simulink library "tbdc"  (Simulink 8.1)
settings: Solver=ode1  StartTime=0.0  StopTime=Inf  FixedStep=0.001  RelTol=1e-3
PostLoadFcn:
  | , if any(exist('dsrtsu_mdlpostloadfcn', 'file') == [2, 3, 6]), try dsrtsu_mdlpostloadfcn('Execute', bdroot); catch fprintf('Error in PostLoadFcn (dsrtsu_mdlpostloadfcn) for model "%s":\n %s\n', bdroot, lasterr); end, end,
undefined symbols (not defined in the file or in its folder): ZERO_FLOAT
libraries: hcu_lib x1
settings Model: DSRTSU_INTERNAL_RTI_VER=450  DSRTSU_INTERNAL_RTI_TYPE=rti1401  RTICANMMDATA=struct('GeneralSetupData',struct('modelroot','D:\ELN150201\Phase3\branches\ACC_Experiments\AdasDragon\software\sw_development\arch\app\jud','generalsettings',struct('filesettings',struct('destfolder',struct('Name','RTICANMM_FILES','Check',1),'buildfolder',struct('Name','.','Check',1),'AbsDestfolder',struct('Name','D:\ELN150201\Phase3\branches\ACC_Experiments\AdasDragon\software\sw_development\arch\app\jud\RTICANMM_FILES'),'AbsBuildfolder',struct('Name','D:\ELN150201\Phase3\branches\ACC_Experiments\AdasDragon\software\sw_development\arch\app\jud'))),'options',struct('addpaths',1,'rmpaths',1,'addtrcexclusion',logical(1),'cannavigator',struct('checkmonitoring',0),'show_usrtrc',0,'use_usrtrc',0),'advanced',struct('options',[1 1 1 1 1 1 1 1 1 1 1 1 1 1 1 1 1 1 1 1 1 1 1 1 1 1 1 1 1 1 1 1 1 1 1 1 1 1 1 1 1 1 1 1 1 1 1 1 1 1 1 1 1 1 1 1 1 1 1 1 1 1 1 1 1 1 1 1 1 1 1 1 1 1 1 1 1 1 1 1 1 1 1 1 1 1 1 1 1 1 1 1 1 1 1 1 1 1 1 1]),'MPSetup',{{}},'modelname','tbdc','block','tbdc'))  DSRTSU_INTERNAL_RTIFPGA=40  Creator=tescamilla  LastModifiedBy=AT015555

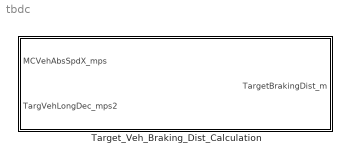
== system tbdc ==
  Target_Veh_Braking_Dist_Calculation : Subsystem

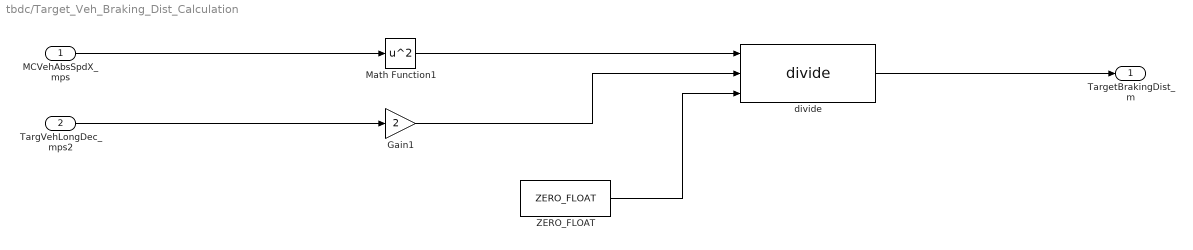
== system tbdc/Target_Veh_Braking_Dist_Calculation ==
  MCVehAbsSpdX_mps : Inport
  TargVehLongDec_mps2 : Inport  Port=2
  Gain1 : Gain  Gain=2
  Math Function1 : Math  Operator=square  SaturateOnIntegerOverflow=on
  ZERO_FLOAT : Constant  Value=ZERO_FLOAT
  divide : hcu_lib/divide
  TargetBrakingDist_m : Outport
  wires:
  TargVehLongDec_mps2/1 -> Gain1/1
  MCVehAbsSpdX_mps/1 -> Math Function1/1
  Gain1/1 -> divide/2
  Math Function1/1 -> divide/1
  divide/1 -> TargetBrakingDist_m/1
  ZERO_FLOAT/1 -> divide/3
